simulink model "cmp_shark_pid2"  (R2022b)
settings: Solver=FixedStepDiscrete  StartTime=0.0  StopTime=3  FixedStep=cmp_Ts  RelTol=1e-3
undefined symbols (not defined in the file or in its folder): cmp_Ts
libraries: slpidlib x1
settings Model: Creator=shark  LastModifiedBy=shark
settings DataIOCC: SaveFormat=Array

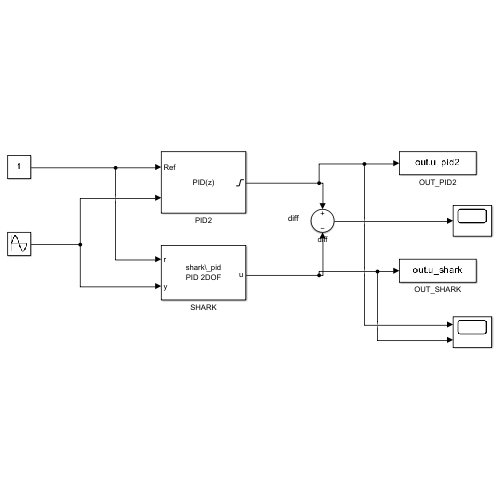
[thumbnail: Simulink's stored preview of the top-level diagram]
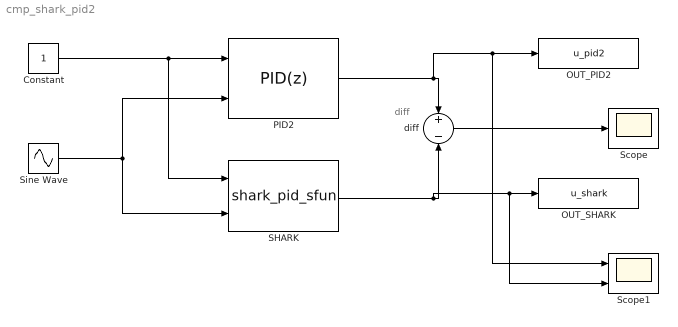
== system cmp_shark_pid2 ==
  note: diff
  Constant : Constant
  OUT_PID2 : ToWorkspace  VariableName=u_pid2  SampleTime=cmp_Ts
  OUT_SHARK : ToWorkspace  VariableName=u_shark  SampleTime=cmp_Ts
  PID2 : slpidlib/PID Controller (2DOF)  Controller=PID  Form=Parallel  TimeDomain=Discrete-time  UseExternalTs=off  SampleTime=0.001  IntegratorMethod=Trapezoidal  FilterMethod=Backward Euler  ControllerParametersSource=internal  P=4  I=1.5  UseKiTs=off  D=0.1  N=50  UseFilter=on  b=1  c=0  TunerSelectOption=Transfer Function Based (PID Tuner App)  InitialConditionSource=internal  InitialConditionForIntegrator=0  InitialConditionForFilter=0  DifferentiatorICPrevScaledInput=0  ExternalReset=none  TrackingMode=off  Kt=1  LimitOutput=on  SatLimitsSource=internal  UpperSaturationLimit=1000000  LowerSaturationLimit=-1000000  LinearizeAsGain=on  AntiWindupMode=clamping  Kb=1  LimitIntegrator=on  UpperIntegratorSaturationLimit=1000000  LowerIntegratorSaturationLimit=-1000000  POutMin=[]  POutMax=[]  IOutMin=[]  IOutMax=[]  DOutMin=[]  DOutMax=[]  NOutMin=[]  NOutMax=[]  bOutMin=[]  bOutMax=[]  cOutMin=[]  cOutMax=[]  SumOutMin=[]  SumOutMax=[]  SaturationOutMin=[]  SaturationOutMax=[]  PParamMin=[]  PParamMax=[]  IParamMin=[]  IParamMax=[]  DParamMin=[]  DParamMax=[]  NParamMin=[]  NParamMax=[]  bParamMin=[]  bParamMax=[]  cParamMin=[]  cParamMax=[]  KbParamMin=[]  KbParamMax=[]  KtParamMin=[]  KtParamMax=[]  KbOutMin=[]  KbOutMax=[]  KtOutMin=[]  KtOutMax=[]  IntegratorOutMin=[]  IntegratorOutMax=[]  FilterOutMin=[]  FilterOutMax=[]  SumI1OutMin=[]  SumI1OutMax=[]  SumI2OutMin=[]  SumI2OutMax=[]  SumI3OutMin=[]  SumI3OutMax=[]  SumI4OutMin=[]  SumI4OutMax=[]  SumDOutMin=[]  SumDOutMax=[]  Sum1OutMin=[]  Sum1OutMax=[]  Sum2OutMin=[]  Sum2OutMax=[]  Sum3OutMin=[]  Sum3OutMax=[]  DifferentiatorOutMin=[]  DifferentiatorOutMax=[]  FilterDiffOutCoefMin=[]  FilterDiffOutCoefMax=[]  ReciprocalOutMin=[]  ReciprocalOutMax=[]  SumDenOutMin=[]  SumDenOutMax=[]  SumNumOutMin=[]  SumNumOutMax=[]  DivideOutMin=[]  DivideOutMax=[]  UdiffTsProdOutMin=[]  UdiffTsProdOutMax=[]  NTsProdOutMin=[]  NTsProdOutMax=[]  UintegralTsProdOutMin=[]  UintegralTsProdOutMax=[]  UngainTsProdOutMin=[]  UngainTsProdOutMax=[]  ClampingZeroOutDataTypeStr=Inherit: Inherit via back propagation  ClampingZeroOutMin=[]  ClampingZeroOutMax=[]  FilterDenConstantOutDataTypeStr=Inherit: Inherit via back propagation  FilterDenConstantOutMin=[]  FilterDenConstantOutMax=[]  PCopyOutDataTypeStr=Inherit: Inherit via back propagation  PCopyOutMin=[]  PCopyOutMax=[]  NCopyOutDataTypeStr=Inherit: Inherit via back propagation  NCopyOutMin=[]  NCopyOutMax=[]  IntegratorContinuousStateAttributes=''  IntegratorStateMustResolveToSignalObject=off  IntegratorRTWStateStorageClass=Auto  FilterContinuousStateAttributes=''  FilterStateMustResolveToSignalObject=off  FilterRTWStateStorageClass=Auto  ParallelPVariant=InternalParameters  IdealPVariant=Disabled  IVariant=InternalParameters  DVariant=InternalParameters  bVariant=InternalParameters  cVariant=InternalParameters  IntegratorVariant=Discrete  SatVariant=Enabled  AWVariant=DiscClampingParallel  PCopyVariant=Disabled  TRVariant=Disabled  FdbkBlocksVariant=Feedback  IdealPFdbkVariant=Passthrough  SatFdbkVariant=Passthrough  DerivativeFilterVariant=BackwardEulerFilter  NVariant=InternalParameters  NCopyVariant=InternalParameters  FilterICVariant=InternalICsFilter  IntegratorICVariant=InternalICs  ExternalResetVariant=Disabled  TRSumVariant=Passthrough  SumFdbkVariant=Enabled  SumVariant=Sum_PID  TsampFilterVariant=InternalTs  TsampNgainVariant=Passthrough  TsampIntegralVariant=Passthrough  ExternalSaturationOutDataTypeStr=Inherit: Same as second input
  SHARK : S-Function  FunctionName=shark_pid_sfun  Parameters=Ts,kp,ki,kd,b,c,n,out_min,out_max,i_min,i_max,imethod-1,awmethod-1,kb  SFunctionDeploymentMode=off  EnableBusSupport=off  mask(shark_pid){Ts=0.001, kp=4, ki=1.5, kd=0.1, b=1, c=0, n=50, out_min=-1000000, out_max=1000000, i_min=-1000000, i_max=1000000, kb=0, imethod=Trapezoidal, awmethod=clamping}
      mask prompts: Ts "Sample time Ts [s]"; kp "kp  (= P)"; ki "ki  [1/s]  (= I)"; kd "kd  [s]    (= D)"; b "Setpoint weight b  (khau P)"; c "Setpoint weight c  (khau D)"; n "Filter coefficient N [rad/s]  (= o N)"; out_min "Gioi han ngo ra: min"; out_max "Gioi han ngo ra: max"; i_min "Gioi han khau I: min"; i_max "Gioi han khau I: max"; kb "Kb [1/s] (chi dung voi back-calculation)"; imethod "Integrator method"; awmethod "Anti-windup method"
      mask help:
      | Bo dieu khien PID nhung shark_pid 2.0 (loi C99).
      | Tuong duong khoi PID (2DOF) khi:
      |   P=kp  I=ki  D=kd  N=n  b=b  c=c
      |   Filter method = Backward Euler
      mask TypeOptions imethod: Backward Euler | Trapezoidal
      mask TypeOptions awmethod: none | clamping | back-calculation
      mask DialogControl grpGain Prompt: He so / Gains
      mask DialogControl grpLim Prompt: Gioi han / Limits
      mask DialogControl grpMeth Prompt: Phuong phap / Methods
      mask Display:
      | port_label('input',1,'r');
      | port_label('input',2,'y');
      | port_label('output',1,'u');
      | disp(sprintf('shark\\_pid\nPID 2DOF'));
  Scope : Scope
  Scope1 : Scope  NumInputPorts=2
  Sine Wave : Sin  SampleTime=0
  diff : Sum  Inputs=+-
  wires:
  Constant/1 -> SHARK/1, PID2/1
  Sine Wave/1 -> PID2/2, SHARK/2
  PID2/1 -> Scope1/1, OUT_PID2/1, diff/1
  SHARK/1 -> Scope1/2, OUT_SHARK/1, diff/2
  diff/1 -> Scope/1
